simulink model "lab2_01"  (R2022a)
settings: Solver=VariableStepAuto  StartTime=0.0  StopTime=10.0  RelTol=1e-3
settings Model: Creator=Illia  LastModifiedBy=Illia

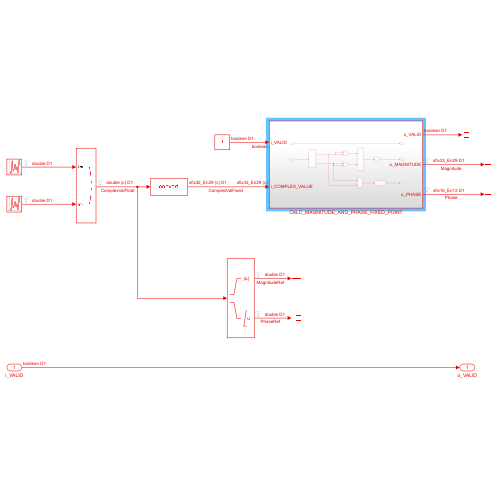
[thumbnail: Simulink's stored preview of the top-level diagram]
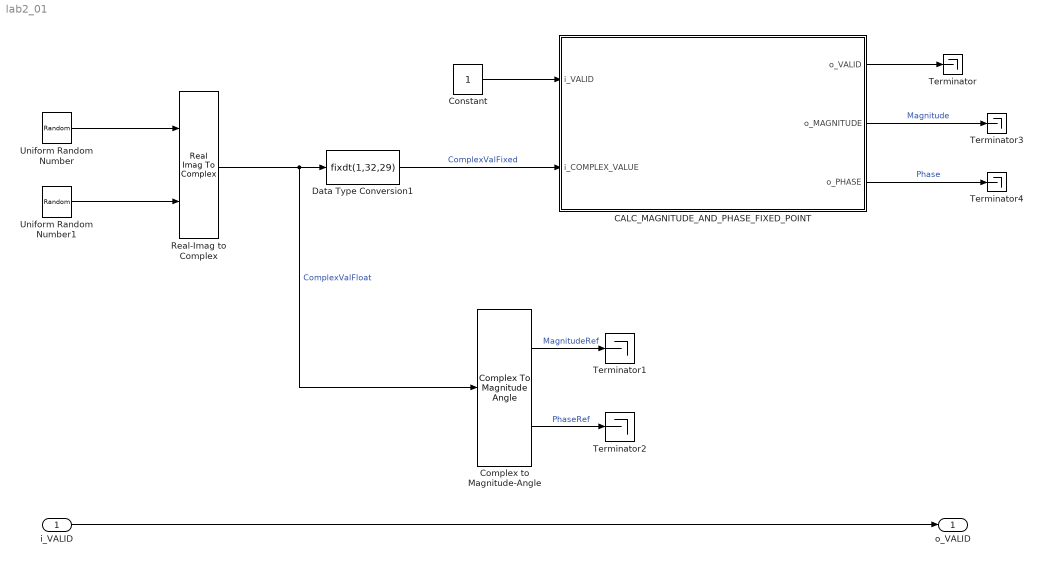
== system lab2_01 ==
  i_VALID : Inport  OutDataTypeStr=boolean
  CALC_MAGNITUDE_AND_PHASE_FIXED_POINT : Subsystem
  Complex to Magnitude-Angle : ComplexToMagnitudeAngle
  Constant : Constant  OutDataTypeStr=boolean  SampleTime=1
  Data Type Conversion1 : DataTypeConversion  OutDataTypeStr=fixdt(1,32,29)  RndMeth=Round  SaturateOnIntegerOverflow=off
  Real-Imag to Complex : RealImagToComplex
  Terminator{,1..4} (5 alike) : Terminator
  Uniform Random Number : UniformRandomNumber  Minimum=-4  Maximum=4  Seed=3  SampleTime=1
  Uniform Random Number1 : UniformRandomNumber  Minimum=-4  Maximum=4  Seed=4  SampleTime=1
  o_VALID : Outport  VectorParamsAs1DForOutWhenUnconnected=off
  wires:
  Uniform Random Number1/1 -> Real-Imag to Complex/2
  Uniform Random Number/1 -> Real-Imag to Complex/1
  Real-Imag to Complex/1 -> Data Type Conversion1/1, Complex to Magnitude-Angle/1  "ComplexValFloat"
  Complex to Magnitude-Angle/1 -> Terminator1/1  "MagnitudeRef"
  Complex to Magnitude-Angle/2 -> Terminator2/1  "PhaseRef"
  Data Type Conversion1/1 -> CALC_MAGNITUDE_AND_PHASE_FIXED_POINT/2(i_COMPLEX_VALUE)  "ComplexValFixed"
  Constant/1 -> CALC_MAGNITUDE_AND_PHASE_FIXED_POINT/1(i_VALID)
  CALC_MAGNITUDE_AND_PHASE_FIXED_POINT/1(o_VALID) -> Terminator/1
  CALC_MAGNITUDE_AND_PHASE_FIXED_POINT/3(o_PHASE) -> Terminator4/1  "Phase"
  CALC_MAGNITUDE_AND_PHASE_FIXED_POINT/2(o_MAGNITUDE) -> Terminator3/1  "Magnitude"
  i_VALID/1 -> o_VALID/1

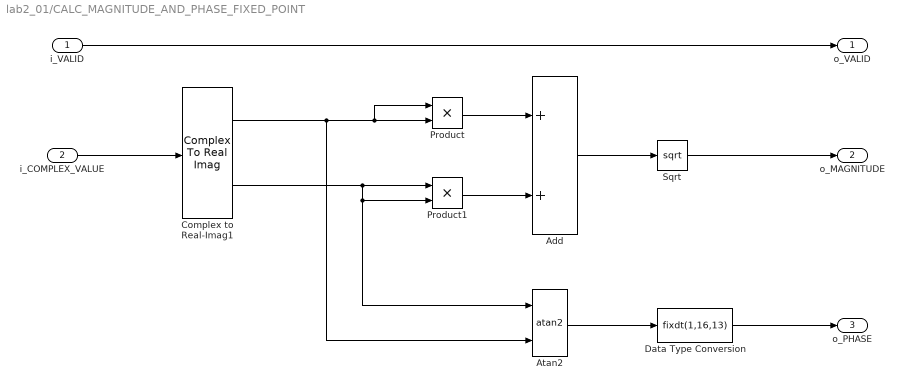
== system lab2_01/CALC_MAGNITUDE_AND_PHASE_FIXED_POINT ==
  i_VALID : Inport  OutDataTypeStr=boolean
  i_COMPLEX_VALUE : Inport  Port=2  OutDataTypeStr=fixdt(1,32,29)
  Add : Sum
  Atan2 : Trigonometry  Operator=atan2  ApproximationMethod=CORDIC
  Complex to Real-Imag1 : ComplexToRealImag
  Data Type Conversion : DataTypeConversion  OutDataTypeStr=fixdt(1,16,13)  RndMeth=Round  SaturateOnIntegerOverflow=off
  Product : Product
  Product1 : Product
  Sqrt : Sqrt  OutDataTypeStr=fixdt(1,33,29)
  o_VALID : Outport  VectorParamsAs1DForOutWhenUnconnected=off
  o_MAGNITUDE : Outport  Port=2  OutDataTypeStr=fixdt(1,33,29)
  o_PHASE : Outport  Port=3  OutDataTypeStr=fixdt(1,16,13)
  wires:
  i_COMPLEX_VALUE/1 -> Complex to Real-Imag1/1
  i_VALID/1 -> o_VALID/1
  Complex to Real-Imag1/1 -> Atan2/2, Product/1, Product/2
  Complex to Real-Imag1/2 -> Product1/1, Product1/2, Atan2/1
  Product1/1 -> Add/2
  Product/1 -> Add/1
  Add/1 -> Sqrt/1
  Sqrt/1 -> o_MAGNITUDE/1
  Atan2/1 -> Data Type Conversion/1
  Data Type Conversion/1 -> o_PHASE/1
